simulink model "ver_2015a"  (R2015a)
settings: Solver=ode45  SolverMode=SingleTasking  StartTime=0.0  StopTime=1000  FixedStep=0.01  MaxStep=1  RelTol=1e-3
values from neighbouring files (symbols this model uses):
  A = [-0.026014706155  0  0; 0.032019398003  -0.0381052395202  0; 0  0.0262404235325  -0.0208551931358]    [matrix_A.mat]
  alpha1 = x1_val(2)    [Zbiorniki.m]    (also in c_table.mat = 0.278702458398; x0_table.mat = 0.278702458398)
  alpha2 = x2_val(2)    [Zbiorniki.m]    (also in c_table.mat = 0.328939614245; x0_table.mat = 0.328939614245)
  alpha3 = x3_val(2)    [Zbiorniki.m]    (also in c_table.mat = 0.404471667446; x0_table.mat = 0.404471667446)
  B = [4.13177021749 0 0]    [matrix_B.mat]
  C = eye(3)    [wywolanie_new.m]
  c1 = x1_val(1)    [Zbiorniki.m]    (also in c_table.mat = 41.0862215805; parametry.mat = 44.608; x0_table.mat = 41.0862215805)
  c2 = x2_val(1)    [Zbiorniki.m]    (also in c_table.mat = 36.7397635112; parametry.mat = 38.7996; x0_table.mat = 36.7397635112)
  c3 = x3_val(1)    [Zbiorniki.m]    (also in c_table.mat = 25.9394235455; parametry.mat = 39.9059; x0_table.mat = 25.9394235455)
  K = lqr(A, B, Q, R)    [wywolanie_new.m]
  L = lqe(A,G,C,Q,R)    [wywolanie_new.m]
undefined symbols (not defined in the file or in its folder): ur, x1r, x2r, x3r
settings Model: CovHtmlReporting=off  Creator=Student  LastModifiedBy=Student

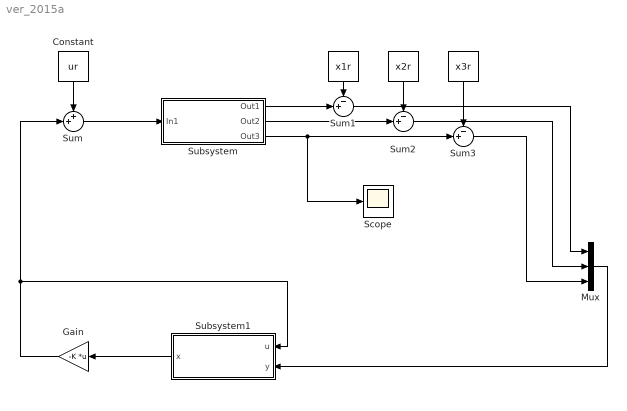
== system ver_2015a ==
  " " : Constant  Value=x2r
  " " : Constant  Value=x1r
  " " : Constant  Value=x3r
  Constant : Constant  Value=ur
  Gain : Gain  Gain=-K  Multiplication=Matrix(K*u)
  Mux : Mux  Inputs=3
  Scope : Scope
      settings: YMin=10.53411  YMax=15.193
  Subsystem : Subsystem
  Subsystem1 : Subsystem
  Sum : Sum  Inputs=++|
  Sum1 : Sum  Inputs=-+|
  Sum2 : Sum  Inputs=-+|
  Sum3 : Sum  Inputs=-+|
  wires:
  Subsystem1/1(x) -> Gain/1
  Gain/1 -> Subsystem1/1("u "), Sum/2
  " "/1 -> Sum1/1
  Constant/1 -> Sum/1
  " "/1 -> Sum2/1
  " "/1 -> Sum3/1
  Sum2/1 -> Mux/2
  Sum3/1 -> Mux/3
  Sum1/1 -> Mux/1
  Mux/1 -> Subsystem1/2("y ")
  Sum/1 -> Subsystem/1(In1)
  Subsystem/1(Out1) -> Sum1/2
  Subsystem/2(Out2) -> Sum2/2
  Subsystem/3(Out3) -> Scope/1, Sum3/2

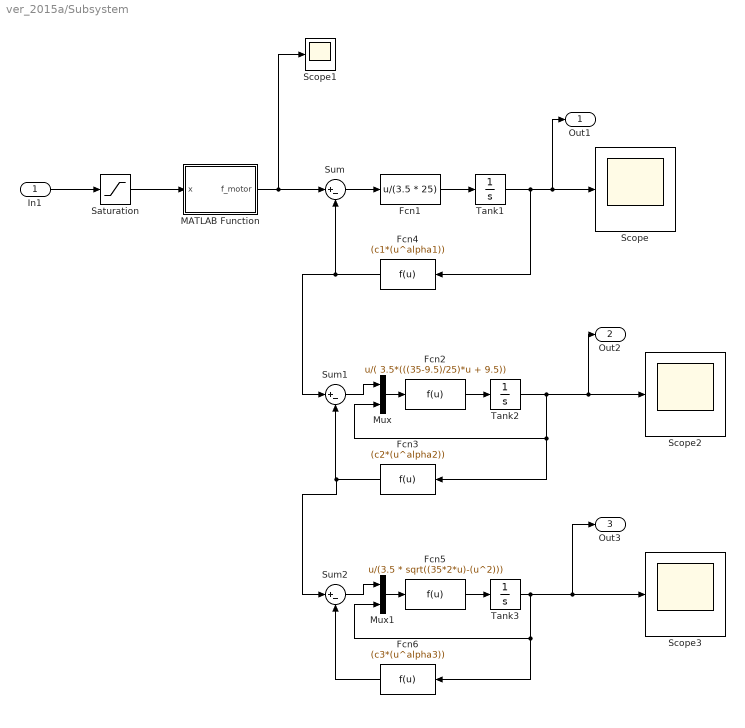
== system ver_2015a/Subsystem ==
  In1 : Inport
  Fcn1 : Fcn  Expr=u/(3.5 * 25)
  Fcn2 : Fcn  Expr=u/( 3.5*(((35-9.5)/25)*u + 9.5))
  Fcn3 : Fcn  Expr=(c2*(u^alpha2))
  Fcn4 : Fcn  Expr=(c1*(u^alpha1))
  Fcn5 : Fcn  Expr=u/(3.5 * sqrt((35*2*u)-(u^2)))
  Fcn6 : Fcn  Expr=(c3*(u^alpha3))
  MATLAB Function : MATLAB Function  TreatAsAtomicUnit=on
  Mux : Mux  Inputs=2
  Mux1 : Mux  Inputs=2
  Saturation : Saturate  UpperLimit=1  LowerLimit=0.5
  Scope{,1..3} (4 alike) : Scope
      Scope1 settings: SaveName=ScopeData4
      Scope2 settings: SaveName=ScopeData2
      Scope3 settings: SaveName=ScopeData3
  Sum : Sum  Inputs=|+-
  Sum1 : Sum  Inputs=|+-
  Sum2 : Sum  Inputs=|+-
  Tank1 : Integrator  InitialCondition=0.1  LimitOutput=on  LowerSaturationLimit=0.1
  Tank2 : Integrator  InitialCondition=0.1  LimitOutput=on  LowerSaturationLimit=0.1
  Tank3 : Integrator  InitialCondition=0.1  LimitOutput=on  LowerSaturationLimit=0.1
  Out1 : Outport
  Out2 : Outport  Port=2
  Out3 : Outport  Port=3
  wires:
  Saturation/1 -> MATLAB Function/1(x)
  In1/1 -> Saturation/1
  MATLAB Function/1(f_motor) -> Scope1/1, Sum/1
  Sum/1 -> Fcn1/1
  Fcn1/1 -> Tank1/1
  Tank1/1 -> Fcn4/1, Out1/1, Scope/1
  Fcn4/1 -> Sum1/1, Sum/2
  Fcn2/1 -> Tank2/1
  Tank2/1 -> Mux/2, Fcn3/1, Out2/1, Scope2/1
  Fcn3/1 -> Sum2/1, Sum1/2
  Mux/1 -> Fcn2/1
  Sum1/1 -> Mux/1
  Fcn5/1 -> Tank3/1
  Tank3/1 -> Out3/1, Scope3/1, Mux1/2, Fcn6/1
  Fcn6/1 -> Sum2/2
  Mux1/1 -> Fcn5/1
  Sum2/1 -> Mux1/1

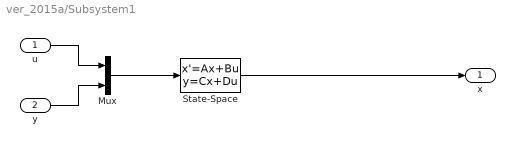
== system ver_2015a/Subsystem1 ==
  "u " : Inport
  "y " : Inport  Port=2
  Mux : Mux  Inputs=2
  State-Space : StateSpace  A=A-L*C  B=[B L]  C=eye(3)  D=zeros(3,4)  X0=zeros(3,1)
  x : Outport
  wires:
  "u "/1 -> Mux/1
  "y "/1 -> Mux/2
  Mux/1 -> State-Space/1
  State-Space/1 -> x/1

== matlab function ver_2015a/Subsystem/MATLAB Function ==
  data: x input; f_motor output
function f_motor = fcn(x)

a1_motor = 4.336406289988628e+02;
a2_motor = -1.346640151767827e+03;
a3_motor = 1.555231837686545e+03;
a4_motor = -5.004734794411548e+02;

f_motor = a1_motor * x^3 + a2_motor * x^2 + a3_motor * x + a4_motor;
